simulink model "schem_1"  (R2024a)
settings: Solver=FixedStepAuto  StartTime=0.0  StopTime=10  FixedStep=1  RelTol=1e-3
undefined symbols (not defined in the file): f1, f2
settings Model: Creator=user  LastModifiedBy=user

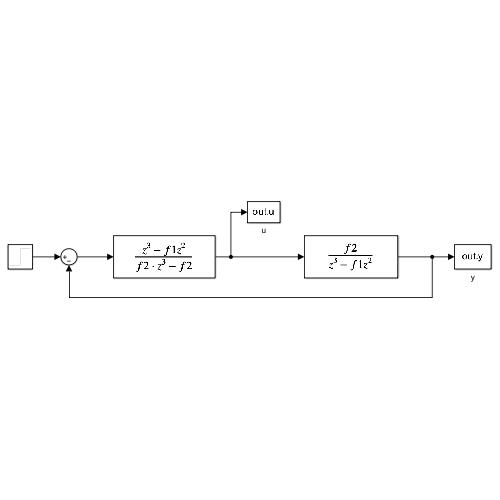
[thumbnail: Simulink's stored preview of the top-level diagram]
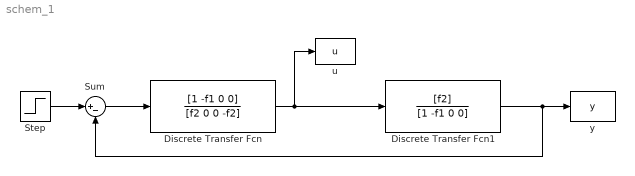
== system schem_1 ==
  Discrete Transfer Fcn : DiscreteTransferFcn  Numerator=[1 -f1 0 0]  Denominator=[f2 0 0 -f2]
  Discrete Transfer Fcn1 : DiscreteTransferFcn  Numerator=[f2]  Denominator=[1 -f1 0 0]
  Step : Step  Time=0  SampleTime=0
  Sum : Sum  Inputs=|+-
  u : ToWorkspace  VariableName=u  SaveFormat=Timeseries  SampleTime=-1
  y : ToWorkspace  VariableName=y  SaveFormat=Timeseries  SampleTime=-1
  wires:
  Discrete Transfer Fcn/1 -> Discrete Transfer Fcn1/1, u/1
  Discrete Transfer Fcn1/1 -> y/1, Sum/2
  Step/1 -> Sum/1
  Sum/1 -> Discrete Transfer Fcn/1
